simulink model "SimulationEnv"  (R2023b)
settings: Solver=VariableStepAuto  StartTime=0.0  StopTime=t_end  RelTol=1e-3
values from neighbouring files (symbols this model uses):
  h = drone.h    [simulate.m]
undefined symbols (not defined in the file or in its folder): A, act_mat, B, C, drone, L, world
libraries: matrix_library x2
settings Model: PacingRate=1000  Creator=HP  LastModifiedBy=HP
settings OptimizationCC: ReuseModelBlockBuffer=off
settings DebuggingCC: AlgebraicLoopMsg=none  ArtificialAlgebraicLoopMsg=none
settings ModelReferenceCC: ModelReferenceMinAlgLoopOccurrences=on

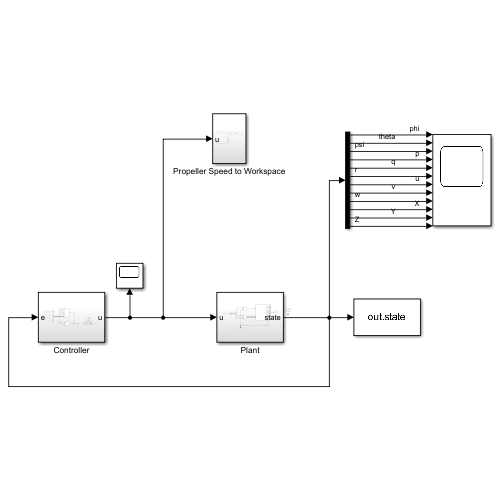
[thumbnail: Simulink's stored preview of the top-level diagram]
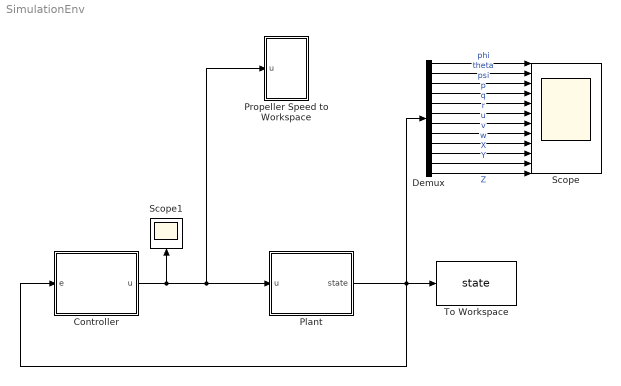
== system SimulationEnv ==
  Controller : Subsystem
  Demux : Demux  Outputs=12
  Plant : Subsystem
  Propeller Speed to Workspace : Subsystem
  Scope : Scope  NumInputPorts=12
  Scope1 : Scope
  To Workspace : ToWorkspace  VariableName=state  SaveFormat=Timeseries  SampleTime=-1
  wires:
  Demux/1 -> Scope/1  "phi"
  Demux/2 -> Scope/2  "theta"
  Demux/3 -> Scope/3  "psi"
  Demux/4 -> Scope/4  "p"
  Demux/5 -> Scope/5  "q"
  Demux/6 -> Scope/6  "r"
  Demux/7 -> Scope/7  "u"
  Demux/8 -> Scope/8  "v"
  Demux/9 -> Scope/9  "w"
  Demux/10 -> Scope/10  "X"
  Demux/11 -> Scope/11  "Y"
  Demux/12 -> Scope/12  "Z"
  Controller/1(u) -> Plant/1(u), Propeller Speed to Workspace/1(u), Scope1/1
  Plant/1(state) -> To Workspace/1, Demux/1, Controller/1(e)

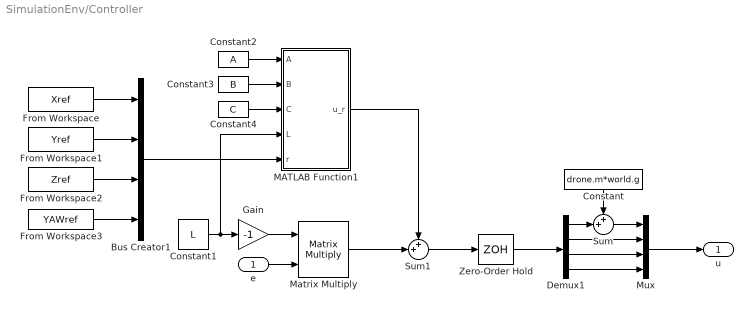
== system SimulationEnv/Controller ==
  e : Inport
  Bus Creator1 : BusCreator  Inputs=4
  Constant : Constant  Value=drone.m*world.g
  Constant1 : Constant  Value=L
  Constant2 : Constant  Value=A
  Constant3 : Constant  Value=B
  Constant4 : Constant  Value=C
  Demux1 : Demux
  From Workspace : FromWorkspace  VariableName=Xref
  From Workspace1 : FromWorkspace  VariableName=Yref
  From Workspace2 : FromWorkspace  VariableName=Zref
  From Workspace3 : FromWorkspace  VariableName=YAWref
  Gain : Gain  Gain=-1
  MATLAB Function1 : MATLAB Function  TreatAsAtomicUnit=on
  Matrix Multiply : Product  Multiplication=Matrix(*)
  Mux : Mux
  Sum : Sum  Inputs=++|
  Sum1 : Sum  Inputs=++|
  Zero-Order Hold : ZeroOrderHold  SampleTime=h
  u : Outport
  wires:
  Demux1/3 -> Mux/3
  Demux1/2 -> Mux/2
  Demux1/4 -> Mux/4
  Demux1/1 -> Sum/2
  Sum/1 -> Mux/1
  Constant/1 -> Sum/1
  Zero-Order Hold/1 -> Demux1/1
  e/1 -> Matrix Multiply/2
  Gain/1 -> Matrix Multiply/1
  Mux/1 -> u/1
  Constant4/1 -> MATLAB Function1/3(C)
  Constant3/1 -> MATLAB Function1/2(B)
  Constant1/1 -> Gain/1, MATLAB Function1/4(L)
  Constant2/1 -> MATLAB Function1/1(A)
  From Workspace3/1 -> Bus Creator1/4
  From Workspace/1 -> Bus Creator1/1
  From Workspace1/1 -> Bus Creator1/2
  From Workspace2/1 -> Bus Creator1/3
  Bus Creator1/1 -> MATLAB Function1/5(r)
  Matrix Multiply/1 -> Sum1/2
  Sum1/1 -> Zero-Order Hold/1
  MATLAB Function1/1(u_r) -> Sum1/1

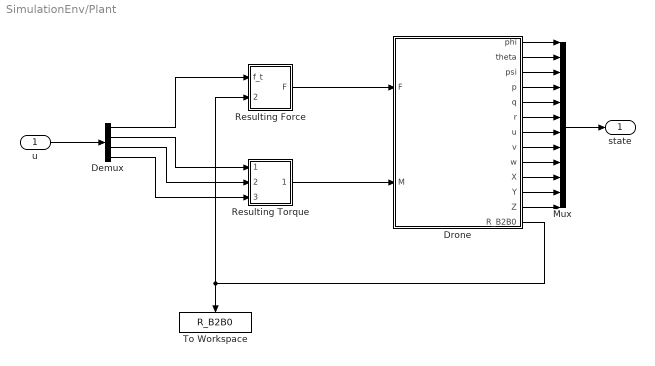
== system SimulationEnv/Plant ==
  u : Inport
  Demux : Demux
  Drone : Subsystem
  Mux : Mux  Inputs=12
  Resulting Force : Subsystem
  Resulting Torque : Subsystem
  To Workspace : ToWorkspace  VariableName=R_B2B0  SampleTime=-1
  state : Outport
  wires:
  Drone/7(u) -> Mux/7
  Drone/2(theta) -> Mux/2
  Drone/4(p) -> Mux/4
  Drone/1(phi) -> Mux/1
  Drone/6(r) -> Mux/6
  Drone/9(w) -> Mux/9
  Demux/4 -> Resulting Torque/3(tau_z)
  Resulting Torque/1(Out1) -> Drone/2(M)
  Drone/5(q) -> Mux/5
  Resulting Force/1(F) -> Drone/1(F)
  Drone/3(psi) -> Mux/3
  Drone/11(Y) -> Mux/11
  Drone/10(X) -> Mux/10
  Drone/8(v) -> Mux/8
  Drone/12(Z) -> Mux/12
  Demux/1 -> Resulting Force/1(f_t)
  Drone/13(R_B2B0) -> Resulting Force/2(R_B2B0), To Workspace/1
  Demux/3 -> Resulting Torque/2(tau_y)
  Demux/2 -> Resulting Torque/1(tau_x)
  u/1 -> Demux/1
  Mux/1 -> state/1

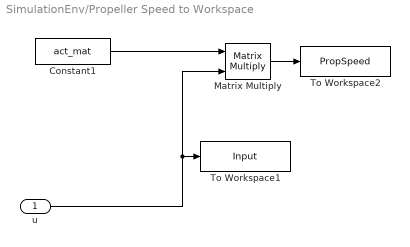
== system SimulationEnv/Propeller Speed to Workspace ==
  u : Inport
  Constant1 : Constant  Value=act_mat
  Matrix Multiply : Product  Multiplication=Matrix(*)
  To Workspace1 : ToWorkspace  VariableName=Input  SaveFormat=Timeseries  SampleTime=-1
  To Workspace2 : ToWorkspace  VariableName=PropSpeed  SaveFormat=Timeseries  SampleTime=-1
  wires:
  Matrix Multiply/1 -> To Workspace2/1
  u/1 -> Matrix Multiply/2, To Workspace1/1
  Constant1/1 -> Matrix Multiply/1

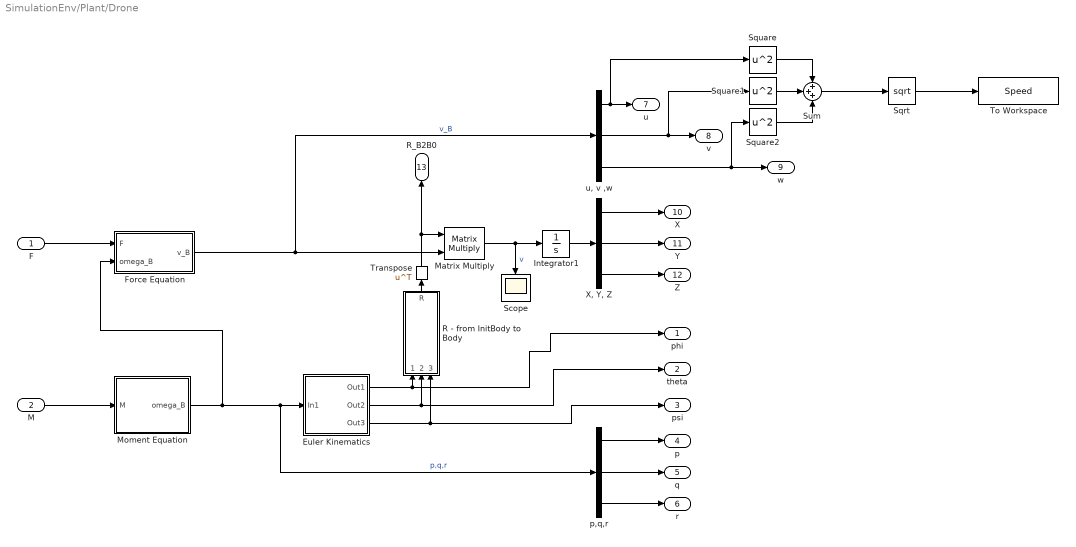
== system SimulationEnv/Plant/Drone ==
  F : Inport
  M : Inport  Port=2
  Euler Kinematics : Subsystem
  Force Equation : Subsystem
  Integrator1 : Integrator  InitialCondition=drone.x0(10:12)
  Matrix Multiply : Product  Multiplication=Matrix(*)
  Moment Equation : Subsystem
  R - from InitBody to Body : MATLAB Function  TreatAsAtomicUnit=on
  Scope : Scope
  Sqrt : Sqrt
  Square : Math  Operator=square
  Square1 : Math  Operator=square
  Square2 : Math  Operator=square
  Sum : Sum  Inputs=+++
  To Workspace : ToWorkspace  VariableName=Speed  SaveFormat=Timeseries  SampleTime=-1
  Transpose : Math  Operator=transpose
  "X, Y, Z" : Demux  Outputs=3
  p,q,r : Demux  Outputs=3
  "u, v ,w" : Demux  Outputs=3
  phi : Outport
  theta : Outport  Port=2
  psi : Outport  Port=3
  p : Outport  Port=4
  q : Outport  Port=5
  r : Outport  Port=6
  u : Outport  Port=7
  v : Outport  Port=8
  w : Outport  Port=9
  X : Outport  Port=10
  Y : Outport  Port=11
  Z : Outport  Port=12
  R_B2B0 : Outport  Port=13
  wires:
  Force Equation/1(v_B) -> Matrix Multiply/2, "u, v ,w"/1  "v_B"
  Euler Kinematics/2(Out2) -> R - from InitBody to Body/2(theta), theta/1
  Euler Kinematics/3(Out3) -> psi/1, R - from InitBody to Body/3(psi)
  "u, v ,w"/2 -> Square1/1, v/1
  "X, Y, Z"/1 -> X/1
  Integrator1/1 -> "X, Y, Z"/1
  Moment Equation/1(omega_B) -> p,q,r/1, Euler Kinematics/1(In1), Force Equation/2(omega_B)  "p,q,r"
  Euler Kinematics/1(Out1) -> R - from InitBody to Body/1(phi), phi/1
  "X, Y, Z"/2 -> Y/1
  Matrix Multiply/1 -> Integrator1/1, Scope/1  "v"
  F/1 -> Force Equation/1(F)
  "X, Y, Z"/3 -> Z/1
  M/1 -> Moment Equation/1(M)
  "u, v ,w"/3 -> Square2/1, w/1
  "u, v ,w"/1 -> Square/1, u/1
  p,q,r/2 -> q/1
  p,q,r/1 -> p/1
  p,q,r/3 -> r/1
  R - from InitBody to Body/1(R) -> Transpose/1
  Transpose/1 -> Matrix Multiply/1, R_B2B0/1
  Square/1 -> Sum/1
  Square1/1 -> Sum/2
  Square2/1 -> Sum/3
  Sum/1 -> Sqrt/1
  Sqrt/1 -> To Workspace/1

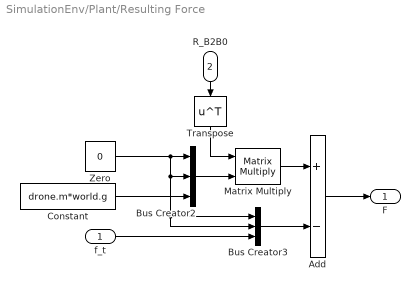
== system SimulationEnv/Plant/Resulting Force ==
  f_t : Inport
  R_B2B0 : Inport  Port=2
  Add : Sum  Inputs=+-
  Bus Creator2 : BusCreator  Inputs=3
  Bus Creator3 : BusCreator  Inputs=3
  Constant : Constant  Value=drone.m*world.g
  Matrix Multiply : Product  Multiplication=Matrix(*)
  Transpose : Math  Operator=transpose
  Zero : Constant  Value=0  OutDataTypeStr=Inherit: Inherit via back propagation
  F : Outport
  wires:
  Bus Creator2/1 -> Matrix Multiply/2
  Add/1 -> F/1
  Zero/1 -> Bus Creator2/2, Bus Creator3/1, Bus Creator3/2, Bus Creator2/1
  R_B2B0/1 -> Transpose/1
  Constant/1 -> Bus Creator2/3
  Transpose/1 -> Matrix Multiply/1
  f_t/1 -> Bus Creator3/3
  Matrix Multiply/1 -> Add/1
  Bus Creator3/1 -> Add/2

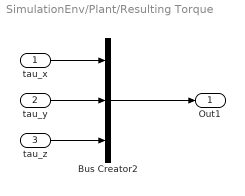
== system SimulationEnv/Plant/Resulting Torque ==
  tau_x : Inport
  tau_y : Inport  Port=2
  tau_z : Inport  Port=3
  Bus Creator2 : BusCreator  Inputs=3
  Out1 : Outport
  wires:
  tau_z/1 -> Bus Creator2/3
  Bus Creator2/1 -> Out1/1
  tau_x/1 -> Bus Creator2/1
  tau_y/1 -> Bus Creator2/2

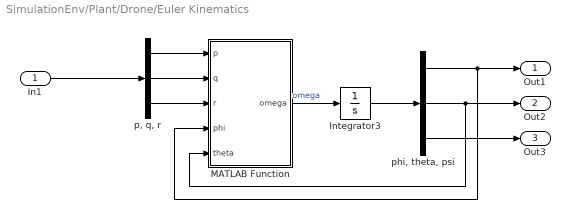
== system SimulationEnv/Plant/Drone/Euler Kinematics ==
  In1 : Inport
  Integrator3 : Integrator  InitialCondition=drone.x0(1:3)
  MATLAB Function : MATLAB Function  TreatAsAtomicUnit=on
  "p, q, r" : Demux  Outputs=3
  "phi, theta, psi" : Demux  Outputs=3
  Out1 : Outport
  Out2 : Outport  Port=2
  Out3 : Outport  Port=3
  wires:
  Integrator3/1 -> "phi, theta, psi"/1
  "p, q, r"/3 -> MATLAB Function/3(r)
  "phi, theta, psi"/2 -> Out2/1, MATLAB Function/5(theta)
  In1/1 -> "p, q, r"/1
  MATLAB Function/1(omega) -> Integrator3/1  "omega"
  "p, q, r"/2 -> MATLAB Function/2(q)
  "phi, theta, psi"/1 -> Out1/1, MATLAB Function/4(phi)
  "p, q, r"/1 -> MATLAB Function/1(p)
  "phi, theta, psi"/3 -> Out3/1

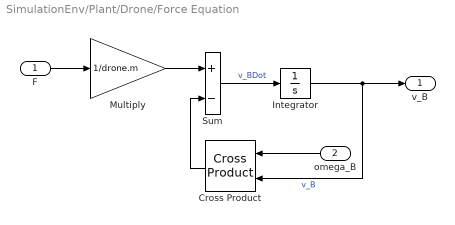
== system SimulationEnv/Plant/Drone/Force Equation ==
  F : Inport
  omega_B : Inport  Port=2
  Cross Product : matrix_library/Cross Product
  Integrator : Integrator  InitialCondition=drone.x0(7:9)
  Multiply : Gain  Gain=1/drone.m
  Sum : Sum  Inputs=+-
  v_B : Outport
  wires:
  Sum/1 -> Integrator/1  "v_BDot"
  Cross Product/1 -> Sum/2
  Integrator/1 -> v_B/1, Cross Product/2  "v_B"
  Multiply/1 -> Sum/1
  F/1 -> Multiply/1
  omega_B/1 -> Cross Product/1

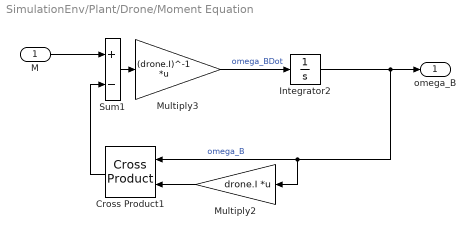
== system SimulationEnv/Plant/Drone/Moment Equation ==
  M : Inport
  Cross Product1 : matrix_library/Cross Product
  Integrator2 : Integrator  InitialCondition=drone.x0(4:6)
  Multiply2 : Gain  Gain=drone.I  Multiplication=Matrix(K*u)
  Multiply3 : Gain  Gain=(drone.I)^-1  Multiplication=Matrix(K*u)
  Sum1 : Sum  Inputs=+-
  omega_B : Outport
  wires:
  Cross Product1/1 -> Sum1/2
  M/1 -> Sum1/1
  Multiply2/1 -> Cross Product1/2
  Multiply3/1 -> Integrator2/1  "omega_BDot"
  Sum1/1 -> Multiply3/1
  Integrator2/1 -> Multiply2/1, Cross Product1/1, omega_B/1  "omega_B"

== matlab function SimulationEnv/Plant/Drone/R - from InitBody to Body ==
  data: phi input; R output; theta input; psi input
function R = B02B(phi, theta, psi)

R = [cos(theta)*cos(psi),   sin(phi)*sin(theta)*cos(psi) - cos(phi)*sin(psi),   cos(phi)*sin(theta)*cos(psi)+sin(phi)*sin(psi);
     cos(theta)*sin(psi),   sin(phi)*sin(theta)*sin(psi) + cos(phi)*cos(psi),   cos(phi)*sin(theta)*sin(psi)-sin(phi)*cos(psi);
     -sin(theta)        ,   sin(phi)*cos(theta)                             ,   cos(phi)*cos(theta)                           ]';

== matlab function SimulationEnv/Plant/Drone/Euler Kinematics/MATLAB Function ==
  data: p input; omega output; q input; r input; phi input; theta input
function omega = fcn(p,q,r, phi, theta)

% T = [1,     0           ,   sin(theta);
%      0,     cos(phi)    ,   -sin(phi)*cos(theta);
%      0,     sin(phi)    ,   cos(theta)*cos(phi)];

T_inv = [1,     tan(theta)*sin(phi)     ,   -tan(theta)*cos(phi);
         0,     cos(phi)                ,   sin(phi);
         0,     -sin(phi)/cos(theta)    ,  cos(phi)/cos(theta)];

omega = T_inv*[p;q;r];

== matlab function SimulationEnv/Controller/MATLAB Function1 ==
  data: A input; u_r output; B input; C input; L input; r input
function u_r = fcn(A, B, C, L, r)

l_r = (C*inv(-A+B*L)*B)\eye(12);

u_r = l_r*[0,0,r(4),0,0,0,0,0,0,r(1),r(2),r(3)]';
